simulink model "three_phase_modular_multilevel_converter"  (R2022a)
settings: Solver=ode23s  StartTime=0.0  StopTime=0.5  RelTol=1e-3
libraries: spsIGBTLib x24, spsSeriesRLCBranchLib x21, spsVoltageMeasurementLib x16, spsCurrentMeasurementLib x6, simulink x6, dspstat3 x6, spsDCVoltageSourceLib x2, spspowerguiLib x1
settings Model: Creator=MC  LastModifiedBy=MC

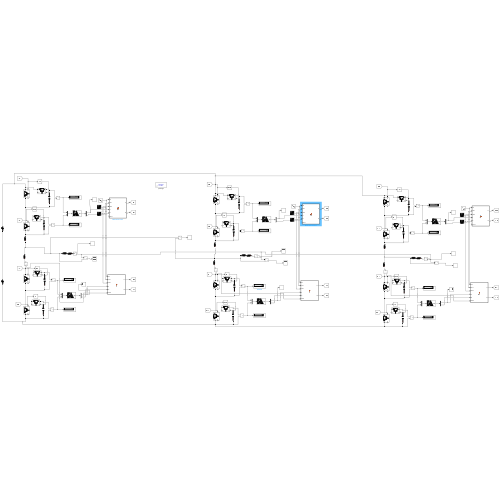
[thumbnail: Simulink's stored preview of the top-level diagram]
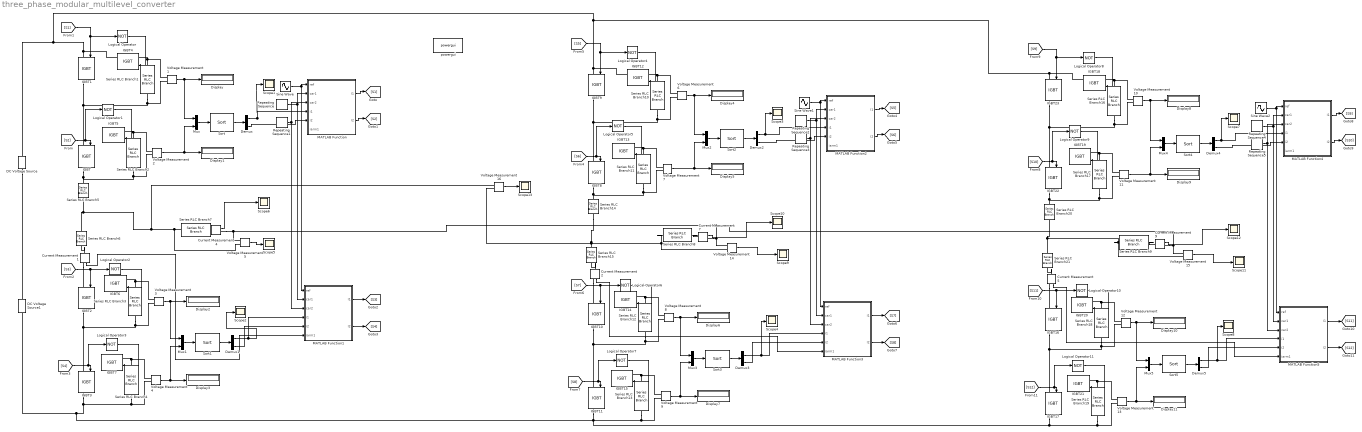
== system three_phase_modular_multilevel_converter ==
  Current Measurement{1..2,4..5,7,9} (6 alike) : spsCurrentMeasurementLib/Current Measurement  PhasorSimulation=off  OutputType=Complex  PSBequivalent=0
  DC Voltage Source : spsDCVoltageSourceLib/DC Voltage Source  Amplitude=100  Measurements=None
  DC Voltage Source1 : spsDCVoltageSourceLib/DC Voltage Source  Amplitude=100  Measurements=None
  Demux{,1..5} (6 alike) : Demux  Outputs=2
  Display{,1..11} (12 alike) : Display
  IGBT{,1..23} (24 alike) : spsIGBTLib/IGBT  Ron=0.001  Lon=0  Vf=1  Tf=1e-6  Tt=2e-6  IC=0  Rs=1e5  Cs=inf  Measurements=on
  Logical Operator{,1..11} (12 alike) : Logic  Operator=NOT  AllPortsSameDT=off  OutDataTypeStr=boolean
  MATLAB Function : MATLAB Function  TreatAsAtomicUnit=on
  MATLAB Function1 : MATLAB Function  TreatAsAtomicUnit=on
  MATLAB Function2 : MATLAB Function  TreatAsAtomicUnit=on
  MATLAB Function3 : MATLAB Function  TreatAsAtomicUnit=on
  MATLAB Function4 : MATLAB Function  TreatAsAtomicUnit=on
  MATLAB Function5 : MATLAB Function  TreatAsAtomicUnit=on
  Mux{,1..5} (6 alike) : Mux  Inputs=2
  Repeating Sequence : simulink/Sources/Repeating Sequence  rep_seq_t=[0 1e-4 2e-4 ]  rep_seq_y=[0 1 0]
  Repeating Sequence1 : simulink/Sources/Repeating Sequence  rep_seq_t=[0 1e-4 2e-4 ]  rep_seq_y=[-1 0 -1]
  Repeating Sequence2 : simulink/Sources/Repeating Sequence  rep_seq_t=[0 1e-4 2e-4 ]  rep_seq_y=[0 1 0]
  Repeating Sequence3 : simulink/Sources/Repeating Sequence  rep_seq_t=[0 1e-4 2e-4 ]  rep_seq_y=[-1 0 -1]
  Repeating Sequence4 : simulink/Sources/Repeating Sequence  rep_seq_t=[0 1e-4 2e-4 ]  rep_seq_y=[0 1 0]
  Repeating Sequence5 : simulink/Sources/Repeating Sequence  rep_seq_t=[0 1e-4 2e-4 ]  rep_seq_y=[-1 0 -1]
  Scope{1..13} (13 alike) : Scope
  Series RLC Branch1 : spsSeriesRLCBranchLib/Series RLC Branch  LConnTagsString=__new0  RConnTagsString=__new0  BranchType=C  Resistance=1  Inductance=1e-3  SetiL0=off  InitialCurrent=0  Capacitance=1000e-6  Setx0=on  InitialVoltage=100  Measurements=None
  Series RLC Branch{2..4,10..13,16..19} (11 alike) : spsSeriesRLCBranchLib/Series RLC Branch  LConnTagsString=__new0  RConnTagsString=__new0  BranchType=C  Resistance=1  Inductance=1e-3  SetiL0=off  InitialCurrent=0  Capacitance=1100e-6  Setx0=on  InitialVoltage=100  Measurements=None
  Series RLC Branch{5..6,14..15,20..21} (6 alike) : spsSeriesRLCBranchLib/Series RLC Branch  LConnTagsString=__new0  RConnTagsString=__new0  BranchType=L  Resistance=1  Inductance=0.01e-3  SetiL0=off  InitialCurrent=0  Capacitance=1100e-6  Setx0=off  InitialVoltage=0  Measurements=None
  Series RLC Branch7 : spsSeriesRLCBranchLib/Series RLC Branch  LConnTagsString=__new0  RConnTagsString=__new0  BranchType=RL  Resistance=1  Inductance=30e-3  SetiL0=off  InitialCurrent=0  Capacitance=1e-6  Setx0=off  InitialVoltage=0  Measurements=None
  Series RLC Branch8 : spsSeriesRLCBranchLib/Series RLC Branch  LConnTagsString=__new0  RConnTagsString=__new0  BranchType=RL  Resistance=1  Inductance=30e-3  SetiL0=off  InitialCurrent=0  Capacitance=1e-6  Setx0=off  InitialVoltage=0  Measurements=None
  Series RLC Branch9 : spsSeriesRLCBranchLib/Series RLC Branch  LConnTagsString=__new0  RConnTagsString=__new0  BranchType=RL  Resistance=1  Inductance=30e-3  SetiL0=off  InitialCurrent=0  Capacitance=1e-6  Setx0=off  InitialVoltage=0  Measurements=None
  Sine Wave : Sin  Amplitude=0.95  Frequency=100*pi  SampleTime=0
  Sine Wave1 : Sin  Amplitude=0.9  Frequency=100*pi  Phase=(-2*pi)/3  SampleTime=0
  Sine Wave2 : Sin  Amplitude=0.9  Frequency=100*pi  Phase=2*pi/3  SampleTime=0
  Sort{,1..5} (6 alike) : dspstat3/Sort  otype=Index  dir=Ascending  sortAlg=Quick sort  roundingMode=Floor  overflowMode=off  accumDataTypeStr=Inherit: Same as product output  accumLastDataTypeStr=Inherit: Same as product output
      settings: SourceProductBaseCode=DS
  Voltage Measurement{1..16} (16 alike) : spsVoltageMeasurementLib/Voltage Measurement  PhasorSimulation=off  OutputType=Complex  PSBequivalent=0
  powergui : spspowerguiLib/powergui  Priority=1  SimulationMode=Discrete  SampleTime=1e-6  frequency=60  Iterations=50  frequencyindice=0  Pbase=100e6  ErrMax=1e-4  UnitsV=kV  UnitsW=MW  buscounter=0  FunctionMessages=off  echomessages=off  EnableUseOfTLC=off  CurrentSourceSwitches=off  DisableSnubberDevices=off  DisableRonSwitches=off  DisableVfSwitches=off  DisplayEquations=off  AutomaticDiscreteSolvers=off  SolverType=Tustin/Backward Euler (TBE)  Interpol=off  ExternalGateDelay=off  methode=off  Ts=100  x0status=blocks  SPID=on  SwTol=0  HookPort=off  NonlinearTolerance=1e-4  nMaxIteration=100  ContinueOnMaxIteration=off  RestoreLinks=warning  ResistiveCurrentMeasurement=off  Frange=[0:2:500]  Ylog=off  Xlog=on  ShowGrid=off  save=off  variable=ZData  structure=0  ZoomFFT=off  StartTime=0.0  cycles=1  DisplayStyle=1  fundamental=60  FreqAxis=off  MaxFrequency=1000  frequencyindicesteady=1  RmsSteady=1  display=off
  wires:
  [S1] -> Logical Operator/1, IGBT1/1
  Sine Wave/1 -> MATLAB Function1/1(ref), MATLAB Function/1(ref)
  Repeating Sequence/1 -> MATLAB Function1/2(car1), MATLAB Function/2(car1)
  Repeating Sequence1/1 -> MATLAB Function1/3(car2), MATLAB Function/3(car2)
  MATLAB Function/1(I1) -> [S1]
  MATLAB Function/2(I2) -> [S2]
  MATLAB Function1/1(I1) -> [S3]
  MATLAB Function1/2(I2) -> [S4]
  Logical Operator/1 -> IGBT4/1
  Voltage Measurement1/1 -> Mux/1, Display/1
  Logical Operator1/1 -> IGBT5/1
  Voltage Measurement2/1 -> Mux/2, Display1/1
  [S2] -> Logical Operator1/1, IGBT/1
  Logical Operator2/1 -> IGBT6/1
  [S3] -> Logical Operator2/1, IGBT2/1
  Logical Operator3/1 -> IGBT7/1
  [S4] -> IGBT3/1, Logical Operator3/1
  Mux/1 -> Sort/1
  Sort/1 -> Demux/1
  Sort1/1 -> Demux1/1
  Voltage Measurement4/1 -> Mux1/2, Display3/1
  Mux1/1 -> Sort1/1
  Voltage Measurement3/1 -> Display2/1, Mux1/1
  Demux/1 -> MATLAB Function/4(i1), Scope1/1
  Demux/2 -> MATLAB Function/5(i2)
  Demux1/2 -> MATLAB Function1/5(i2)
  Current Measurement1/1 -> MATLAB Function1/6(iarm1)
  Demux1/1 -> Scope2/1, MATLAB Function1/4(i1)
  Current Measurement4/1 -> Scope6/1
  Voltage Measurement5/1 -> Scope5/1
  Sort2/1 -> Demux2/1
  Logical Operator7/1 -> IGBT15/1
  Logical Operator5/1 -> IGBT13/1
  Demux2/2 -> MATLAB Function2/5(i2)
  MATLAB Function3/1(I1) -> [S7]
  MATLAB Function2/1(I1) -> [S5]
  Repeating Sequence2/1 -> MATLAB Function3/2(car1), MATLAB Function2/2(car1)
  Voltage Measurement7/1 -> Mux2/2, Display5/1
  Voltage Measurement8/1 -> Display6/1, Mux3/1
  Demux2/1 -> MATLAB Function2/4(i1), Scope3/1
  Repeating Sequence3/1 -> MATLAB Function3/3(car2), MATLAB Function2/3(car2)
  Mux2/1 -> Sort2/1
  MATLAB Function2/2(I2) -> [S6]
  [S7] -> Logical Operator6/1, IGBT10/1
  Voltage Measurement9/1 -> Mux3/2, Display7/1
  MATLAB Function3/2(I2) -> [S8]
  Sort3/1 -> Demux3/1
  Logical Operator6/1 -> IGBT14/1
  [S8] -> IGBT11/1, Logical Operator7/1
  [S6] -> Logical Operator5/1, IGBT8/1
  [S5] -> Logical Operator4/1, IGBT9/1
  Current Measurement2/1 -> MATLAB Function3/6(iarm1)
  Mux3/1 -> Sort3/1
  Sine Wave1/1 -> MATLAB Function3/1(ref), MATLAB Function2/1(ref)
  Logical Operator4/1 -> IGBT12/1
  Demux3/1 -> MATLAB Function3/4(i1), Scope4/1
  Demux3/2 -> MATLAB Function3/5(i2)
  Voltage Measurement6/1 -> Mux2/1, Display4/1
  Logical Operator8/1 -> IGBT18/1
  Sine Wave2/1 -> MATLAB Function5/1(ref), MATLAB Function4/1(ref)
  Voltage Measurement10/1 -> Mux4/1, Display8/1
  Demux5/2 -> MATLAB Function5/5(i2)
  Current Measurement5/1 -> MATLAB Function5/6(iarm1)
  [S10] -> Logical Operator9/1, IGBT22/1
  [S12] -> IGBT17/1, Logical Operator11/1
  Mux5/1 -> Sort5/1
  [S9] -> Logical Operator8/1, IGBT23/1
  Repeating Sequence5/1 -> MATLAB Function5/3(car2), MATLAB Function4/3(car2)
  [S11] -> Logical Operator10/1, IGBT16/1
  Logical Operator10/1 -> IGBT20/1
  Sort5/1 -> Demux5/1
  MATLAB Function4/2(I2) -> [S10]
  Mux4/1 -> Sort4/1
  Voltage Measurement11/1 -> Mux4/2, Display9/1
  Repeating Sequence4/1 -> MATLAB Function5/2(car1), MATLAB Function4/2(car1)
  Voltage Measurement13/1 -> Mux5/2, Display11/1
  Logical Operator11/1 -> IGBT21/1
  Sort4/1 -> Demux4/1
  Demux4/2 -> MATLAB Function4/5(i2)
  Voltage Measurement12/1 -> Display10/1, Mux5/1
  Demux5/1 -> MATLAB Function5/4(i1), Scope8/1
  MATLAB Function4/1(I1) -> [S9]
  MATLAB Function5/2(I2) -> [S12]
  MATLAB Function5/1(I1) -> [S11]
  Logical Operator9/1 -> IGBT19/1
  Demux4/1 -> MATLAB Function4/4(i1), Scope7/1
  Voltage Measurement14/1 -> Scope9/1
  Current Measurement7/1 -> Scope10/1
  Voltage Measurement15/1 -> Scope11/1
  Current Measurement9/1 -> Scope12/1
  Voltage Measurement16/1 -> Scope13/1
  connections:
  Series RLC Branch19/LConn1 -- Voltage Measurement13/LConn2 -- DC Voltage Source1/LConn1 -- IGBT3/RConn1 -- Voltage Measurement4/LConn2 -- Series RLC Branch4/LConn1 -- IGBT11/RConn1 -- Voltage Measurement9/LConn2 -- Series RLC Branch13/LConn1 -- IGBT17/RConn1
  IGBT23/LConn1 -- IGBT4/RConn1 -- IGBT1/LConn1 -- DC Voltage Source/RConn1 -- IGBT12/RConn1 -- IGBT9/LConn1 -- IGBT18/RConn1
  Series RLC Branch3/LConn1 -- Voltage Measurement3/LConn2 -- IGBT2/RConn1 -- IGBT3/LConn1
  DC Voltage Source/LConn1 -- DC Voltage Source1/RConn1
  IGBT1/RConn1 -- Voltage Measurement1/LConn2 -- Series RLC Branch1/LConn1 -- IGBT/LConn1
  Series RLC Branch1/RConn1 -- Voltage Measurement1/LConn1 -- IGBT4/LConn1
  Series RLC Branch2/RConn1 -- Voltage Measurement2/LConn1 -- IGBT5/LConn1
  Series RLC Branch3/RConn1 -- Voltage Measurement3/LConn1 -- IGBT6/LConn1
  Series RLC Branch4/RConn1 -- Voltage Measurement4/LConn1 -- IGBT7/LConn1
  Voltage Measurement2/LConn2 -- Series RLC Branch2/LConn1 -- IGBT/RConn1 -- Series RLC Branch5/RConn1
  Current Measurement1/LConn1 -- Series RLC Branch6/LConn1
  Current Measurement1/RConn1 -- IGBT2/LConn1
  Series RLC Branch5/LConn1 -- Voltage Measurement16/LConn1 -- Voltage Measurement5/LConn2 -- Series RLC Branch7/RConn1 -- Series RLC Branch6/RConn1
  Series RLC Branch7/LConn1 -- Current Measurement4/LConn1
  IGBT11/LConn1 -- Voltage Measurement8/LConn2 -- Series RLC Branch12/LConn1 -- IGBT10/RConn1
  IGBT13/LConn1 -- Voltage Measurement7/LConn1 -- Series RLC Branch11/RConn1
  IGBT8/LConn1 -- Voltage Measurement6/LConn2 -- Series RLC Branch10/LConn1 -- IGBT9/RConn1
  Series RLC Branch14/RConn1 -- IGBT8/RConn1 -- Voltage Measurement7/LConn2 -- Series RLC Branch11/LConn1
  IGBT14/LConn1 -- Voltage Measurement8/LConn1 -- Series RLC Branch12/RConn1
  IGBT15/LConn1 -- Voltage Measurement9/LConn1 -- Series RLC Branch13/RConn1
  IGBT12/LConn1 -- Voltage Measurement6/LConn1 -- Series RLC Branch10/RConn1
  Current Measurement2/LConn1 -- Series RLC Branch15/LConn1
  Current Measurement2/RConn1 -- IGBT10/LConn1
  IGBT18/LConn1 -- Voltage Measurement10/LConn1 -- Series RLC Branch16/RConn1
  IGBT21/LConn1 -- Voltage Measurement13/LConn1 -- Series RLC Branch19/RConn1
  Series RLC Branch20/RConn1 -- IGBT22/RConn1 -- Voltage Measurement11/LConn2 -- Series RLC Branch17/LConn1
  IGBT22/LConn1 -- Voltage Measurement10/LConn2 -- Series RLC Branch16/LConn1 -- IGBT23/RConn1
  IGBT19/LConn1 -- Voltage Measurement11/LConn1 -- Series RLC Branch17/RConn1
  IGBT17/LConn1 -- IGBT16/RConn1 -- Voltage Measurement12/LConn2 -- Series RLC Branch18/LConn1
  IGBT20/LConn1 -- Voltage Measurement12/LConn1 -- Series RLC Branch18/RConn1
  Current Measurement5/LConn1 -- Series RLC Branch21/LConn1
  Current Measurement5/RConn1 -- IGBT16/LConn1
  Current Measurement9/RConn1 -- Voltage Measurement5/LConn1 -- Current Measurement4/RConn1 -- Voltage Measurement14/LConn1 -- Current Measurement7/RConn1 -- Voltage Measurement15/LConn1
  Series RLC Branch8/LConn1 -- Current Measurement7/LConn1
  Series RLC Branch8/RConn1 -- Voltage Measurement16/LConn2 -- Series RLC Branch14/LConn1 -- Series RLC Branch15/RConn1 -- Voltage Measurement14/LConn2
  Series RLC Branch9/LConn1 -- Current Measurement9/LConn1
  Series RLC Branch9/RConn1 -- Voltage Measurement15/LConn2 -- Series RLC Branch21/RConn1 -- Series RLC Branch20/LConn1

== matlab function three_phase_modular_multilevel_converter/MATLAB Function1 ==
  data: ref input; I1 output; car1 input; car2 input; I2 output; i1 input; i2 input; iarm1 input
function [I1,I2] = fcn(ref,car1,car2,i1,i2,iarm1)

 signal= zeros(2,1);
 if ref >= car1
    signal(i1)=0;
    signal(i2)=0;
 elseif ref< car1 && ref> car2
     if iarm1>= 0 
     signal(i1)=0;
     signal(i2)=1;
     else 
     signal(i1)=1;
     signal(i2)=0;
     end
 elseif ref < car2
    signal(i1)=1;
    signal(i2)=1;
 end
 I1=signal(1);
 I2=signal(2);
end

== matlab function three_phase_modular_multilevel_converter/MATLAB Function ==
  data: ref input; I1 output; car1 input; car2 input; I2 output; i1 input; i2 input; iarm1 input
function [I1,I2] = fcn(ref,car1,car2,i1,i2,iarm1)

 signal= zeros(2,1);
 if ref >= car1
    signal(i1)=1;
    signal(i2)=1;
 elseif ref< car1 && ref> car2
     if iarm1>= 0 
     signal(i1)=0;
     signal(i2)=1;
     else 
     signal(i1)=1;
     signal(i2)=0;
     end
 elseif ref < car2
    signal(i1)=0;
    signal(i2)=0;
 end
 I1=signal(1);
 I2=signal(2);
end

== matlab function three_phase_modular_multilevel_converter/MATLAB Function2 ==
  data: ref input; I1 output; car1 input; car2 input; I2 output; i1 input; i2 input; iarm1 input
function [I1,I2] = fcn(ref,car1,car2,i1,i2,iarm1)

 signal= zeros(2,1);
 if ref >= car1
    signal(i1)=1;
    signal(i2)=1;
 elseif ref< car1 && ref> car2
     if iarm1>= 0 
     signal(i1)=0;
     signal(i2)=1;
     else 
     signal(i1)=1;
     signal(i2)=0;
     end
 elseif ref < car2
    signal(i1)=0;
    signal(i2)=0;
 end
 I1=signal(1);
 I2=signal(2);
end

== matlab function three_phase_modular_multilevel_converter/MATLAB Function3 ==
  data: ref input; I1 output; car1 input; car2 input; I2 output; i1 input; i2 input; iarm1 input
function [I1,I2] = fcn(ref,car1,car2,i1,i2,iarm1)

 signal= zeros(2,1);
 if ref >= car1
    signal(i1)=0;
    signal(i2)=0;
 elseif ref< car1 && ref> car2
     if iarm1>= 0 
     signal(i1)=0;
     signal(i2)=1;
     else 
     signal(i1)=1;
     signal(i2)=0;
     end
 elseif ref < car2
    signal(i1)=1;
    signal(i2)=1;
 end
 I1=signal(1);
 I2=signal(2);
end

== matlab function three_phase_modular_multilevel_converter/MATLAB Function4 ==
  data: ref input; I1 output; car1 input; car2 input; I2 output; i1 input; i2 input; iarm1 input
function [I1,I2] = fcn(ref,car1,car2,i1,i2,iarm1)

 signal= zeros(2,1);
 if ref >= car1
    signal(i1)=1;
    signal(i2)=1;
 elseif ref< car1 && ref> car2
     if iarm1>= 0 
     signal(i1)=0;
     signal(i2)=1;
     else 
     signal(i1)=1;
     signal(i2)=0;
     end
 elseif ref < car2
    signal(i1)=0;
    signal(i2)=0;
 end
 I1=signal(1);
 I2=signal(2);
end

== matlab function three_phase_modular_multilevel_converter/MATLAB Function5 ==
  data: ref input; I1 output; car1 input; car2 input; I2 output; i1 input; i2 input; iarm1 input
function [I1,I2] = fcn(ref,car1,car2,i1,i2,iarm1)

 signal= zeros(2,1);
 if ref >= car1
    signal(i1)=0;
    signal(i2)=0;
 elseif ref< car1 && ref> car2
     if iarm1>= 0 
     signal(i1)=0;
     signal(i2)=1;
     else 
     signal(i1)=1;
     signal(i2)=0;
     end
 elseif ref < car2
    signal(i1)=1;
    signal(i2)=1;
 end
 I1=signal(1);
 I2=signal(2);
end
